simulink model "PIDController"  (R2020b)
settings: Solver=VariableStepAuto  StartTime=0.0  StopTime=10.0  RelTol=1e-3
settings Model: Creator=005274  LastModifiedBy=005274

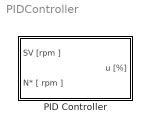
== system PIDController ==
  PID Controller : Subsystem  mask{Kp=0, Ki=0, Kd=0}
      mask prompts: Kp "Proportional"; Ki "Integral"; Kd "Derivative"

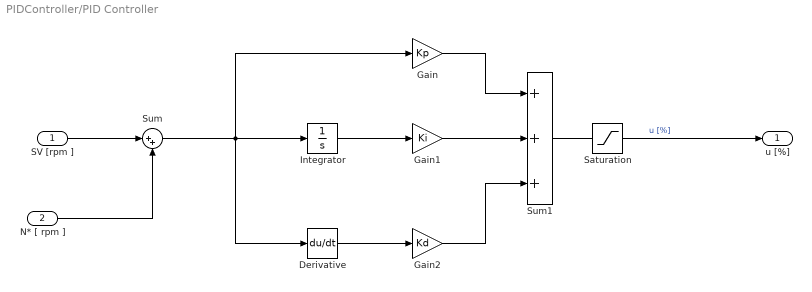
== system PIDController/PID Controller ==
  SV [rpm ] : Inport
  N* [ rpm ] : Inport  Port=2
  Derivative : Derivative
  Gain : Gain  Gain=Kp
  Gain1 : Gain  Gain=Ki
  Gain2 : Gain  Gain=Kd
  Integrator : Integrator
  Saturation : Saturate
  Sum : Sum  Inputs=|++
  Sum1 : Sum  Inputs=+++
  u [%] : Outport
  wires:
  Gain1/1 -> Sum1/2
  Sum/1 -> Gain/1, Integrator/1, Derivative/1
  Sum1/1 -> u [%]/1  "u [%]"
  Gain2/1 -> Sum1/3
  Gain/1 -> Sum1/1
  Derivative/1 -> Gain2/1
  Integrator/1 -> Gain1/1
  N* [ rpm ]/1 -> Sum/2
  SV [rpm ]/1 -> Sum/1
